simulink model "FFT_Model"  (R2013a)
settings: Solver=FixedStepDiscrete  StartTime=0.0  StopTime=.512  FixedStep=Ts  RelTol=1e-3
InitFcn:
  | Ts=1/1000;
undefined symbols (not defined in the file or in its folder): Fs, get
libraries: dspxfrm3 x1, dspsrcs4 x1, dspsnks4 x1, dspsigops x1
settings Model: Creator=Lee  LastModifiedBy=Lee

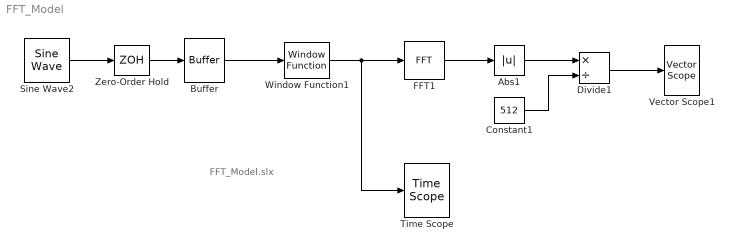
== system FFT_Model ==
  note: FFT_Model.slx
  Abs1 : Abs
  Buffer : Buffer  N=512  TreatMby1Signals=One channel
  Constant1 : Constant  Value=512
  Divide1 : Product  Inputs=*/
  FFT1 : dspxfrm3/FFT  CompMethod=Table lookup  TableOpt=NEW  TableOptActive=Speed  BitRevOrder=off  InheritFFTLength=on  FFTLength=64  RowConvenienceOn=on  FFTImplementation=Auto  SkipNorm=off  firstCoeffDataTypeStr=Inherit: Same word length as input  firstCoeffLastDataTypeStr=Inherit: Same word length as input  outputMin=[]  outputMax=[]  roundingMode=Floor  overflowMode=off
  Sine Wave2 : dspsrcs4/Sine Wave  Amplitude=1  Frequency=100/.512  Phase=0  SampleMode=Continuous  OutComplex=Real  CompMethod=Trigonometric fcn  TableSize=Speed  SampleTime=1/1000  SamplesPerFrame=512  ResetState=Restart at time zero  dataType=double  wordLen=16  udDataType=sfix(16)  fracBitsMode=Best precision  numFracBits=15  OutDataTypeStr=double  LastOutDataTypeStr=double
  Time Scope : TimeScope  DefaultConfigurationName=spbscopes.TimeScopeBlockCfg
      settings: CopyFcn=scopeextensions.ScopeBlock.callback(gcbh, 'onBlockCopy', gcbh);  DeleteFcn=scopeextensions.ScopeBlock.callback(gcbh, 'onBlockDelete');  PreSaveFcn=scopeextensions.ScopeBlock.callback(gcbh, 'onModelSave');  NameChangeFcn=scopeextensions.ScopeBlock.callback(gcbh, 'onBlockRename');  CloseFcn=scopeextensions.ScopeBlock.callback(gcbh, 'onBlockClose');  PreDeleteFcn=scopeextensions.ScopeBlock.callback(gcbh, 'onBlockPreDelete');
  Vector Scope1 : dspsnks4/Vector Scope  ScopeProperties=on  Domain=Frequency  HorizSpan=1  DisplayProperties=off  AxisGrid=on  Memory=off  FrameNumber=on  AxisLegend=off  AxisZoom=off  OpenScopeAtSimStart=on  OpenScopeImmediately=off  FigPos=get(0,'defaultfigureposition')  AxisProperties=off  XUnits=Hertz  XRange=[-Fs/2...Fs/2]  InheritXIncr=on  XIncr=1  XLabel=Time  XLimit=Auto  XMin=0  XMax=1  XStart=0  YUnits=dB  YLabel=Amplitude  LineProperties=off  XAxisParamsVer=6.9
      settings: YMin=-160  YMax=1
  Window Function1 : dspsigops/Window Function  winmode=Apply window to input  wintype=Boxcar  sampmode=Continuous  samptime=1  N=64  Rs=50  beta=10  winsamp=Symmetric  UserWindow=hamming  OptParams=off  UserParams={'symmetric'}  RowConvenienceOn=on  dataType=double  isSigned=on  wordLen=16  udDataType=sfix(16)  fracBitsMode=Best precision  numFracBits=15  roundingMode=Floor  overflowMode=off  numSidelobes=4  sidelobeLevel=-30
  Zero-Order Hold : ZeroOrderHold  SampleTime=Ts
  wires:
  Sine Wave2/1 -> Zero-Order Hold/1
  Zero-Order Hold/1 -> Buffer/1
  FFT1/1 -> Abs1/1
  Constant1/1 -> Divide1/2
  Abs1/1 -> Divide1/1
  Divide1/1 -> Vector Scope1/1
  Buffer/1 -> Window Function1/1
  Window Function1/1 -> FFT1/1, Time Scope/1
